simulink model "ABS"  (R2022b)
settings: Solver=VariableStepAuto  StartTime=0.0  StopTime=25  RelTol=1e-3
model workspace (MAT data in the model file):
  I = 5
  Jw = 0.02
  R = 0.28
  g = 9.81
  m = 75
  rw = 1.25
  v0 = 44
settings Model: Creator=ParkJunHo  LastModifiedBy=ParkJunHo

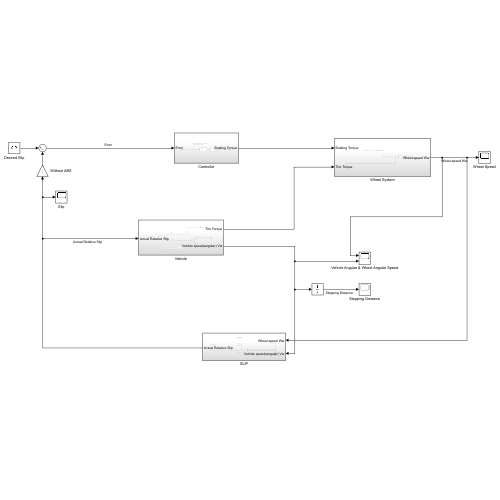
[thumbnail: Simulink's stored preview of the top-level diagram]
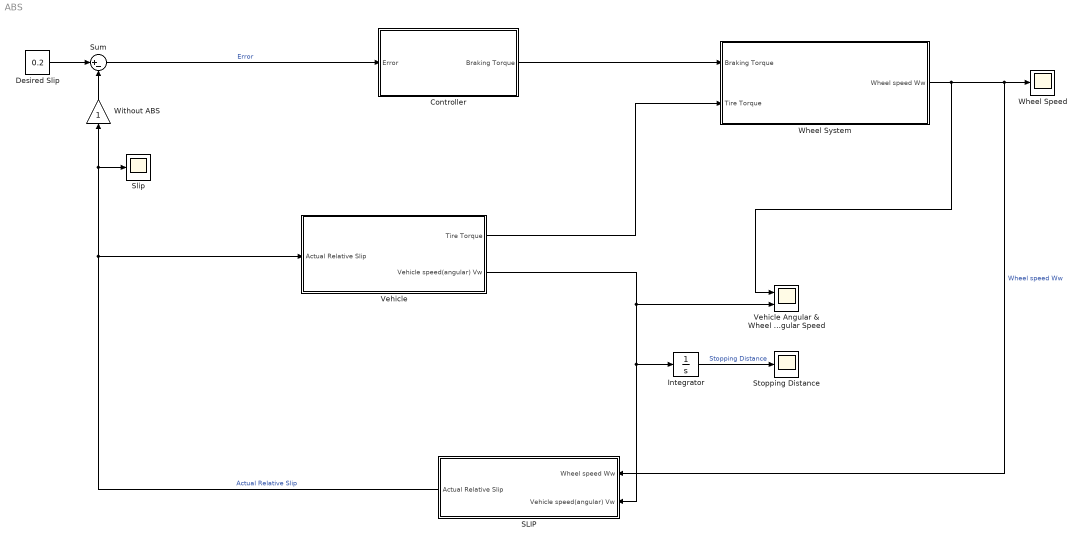
== system ABS ==
  Controller : Subsystem
  Desired Slip : Constant  Value=0.2
  Integrator : Integrator
  SLIP : Subsystem
  Slip : Scope
  Stopping Distance : Scope
  Sum : Sum  Inputs=|+-
  Vehicle : Subsystem
  Vehicle Angular & Wheel Angular Speed : Scope  NumInputPorts=2
  Wheel Speed : Scope
  Wheel System : Subsystem
  Without ABS : Gain
  wires:
  Desired Slip/1 -> Sum/1
  Wheel System/1(Wheel speed Ww) -> Vehicle Angular & Wheel Angular Speed/1, SLIP/1(Wheel speed Ww), Wheel Speed/1  "Wheel speed Ww"
  Sum/1 -> Controller/1(Error)  "Error"
  Controller/1(Braking Torque) -> Wheel System/1(Braking Torque)
  SLIP/1(Actual Relative Slip) -> Without ABS/1, Slip/1, Vehicle/1(Actual Relative Slip)  "Actual Relative Slip"
  Vehicle/1(Tire Torque) -> Wheel System/2(Tire Torque)
  Vehicle/2(Vehicle speed(angular) Vw) -> Vehicle Angular & Wheel Angular Speed/2, Integrator/1, SLIP/2(Vehicle speed(angular) Vw)
  Integrator/1 -> Stopping Distance/1  "Stopping Distance"
  Without ABS/1 -> Sum/2

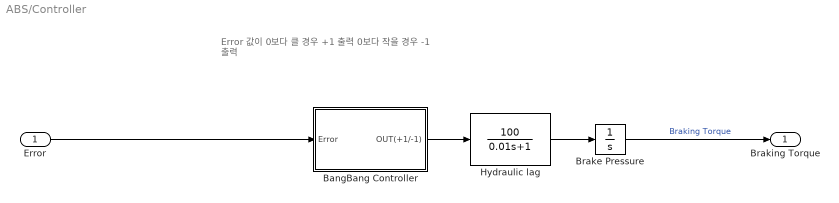
== system ABS/Controller ==
  note: Error 값이 0보다 클 경우 +1 출력
      | 0보다 작을 경우 -1 출력
  Error : Inport
  BangBang Controller : Subsystem
  Brake Pressure : Integrator  LimitOutput=on  UpperSaturationLimit=1000  LowerSaturationLimit=0
  Hydraulic lag : TransferFcn  Numerator=[100]  Denominator=[0.01 1]
  Braking Torque : Outport
  wires:
  BangBang Controller/1(OUT(+1/-1)) -> Hydraulic lag/1
  Hydraulic lag/1 -> Brake Pressure/1
  Error/1 -> BangBang Controller/1(Error)
  Brake Pressure/1 -> Braking Torque/1  "Braking Torque"

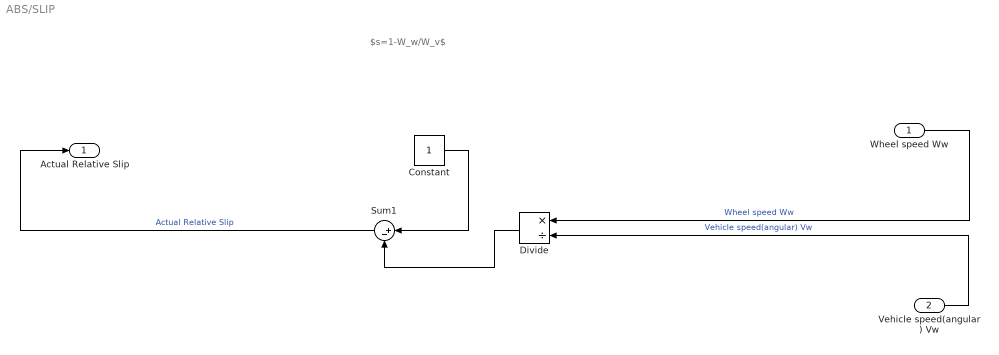
== system ABS/SLIP ==
  note: $s=1-W_w/W_v$
  Wheel speed Ww : Inport
  Vehicle speed(angular) Vw : Inport  Port=2
  Constant : Constant
  Divide : Product  Inputs=*/
  Sum1 : Sum  Inputs=|+-
  Actual Relative Slip : Outport
  wires:
  Divide/1 -> Sum1/2
  Wheel speed Ww/1 -> Divide/1  "Wheel speed Ww"
  Constant/1 -> Sum1/1
  Vehicle speed(angular) Vw/1 -> Divide/2  "Vehicle speed(angular) Vw"
  Sum1/1 -> Actual Relative Slip/1  "Actual Relative Slip"

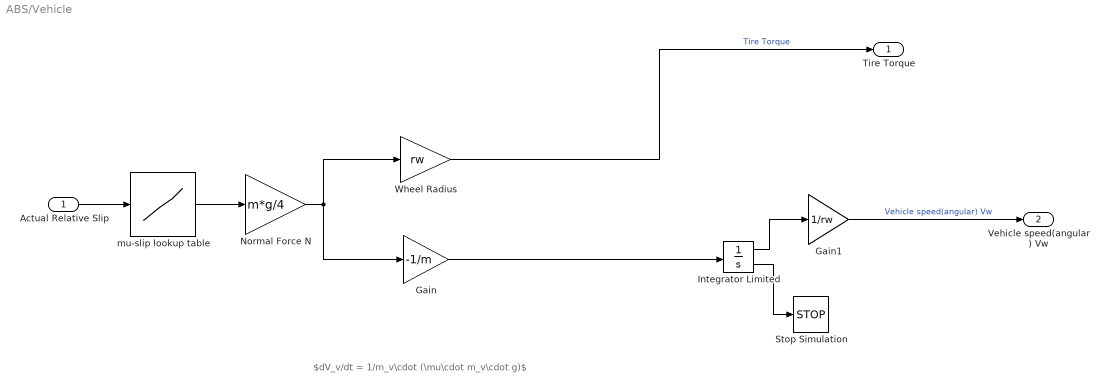
== system ABS/Vehicle ==
  note: $dV_v/dt = 1/m_v\cdot (\mu\cdot m_v\cdot g)$
  Actual Relative Slip : Inport
  Gain : Gain  Gain=-1/m
  Gain1 : Gain  Gain=1/rw
  Integrator Limited : Integrator  InitialCondition=v0  LimitOutput=on  UpperSaturationLimit=1000  LowerSaturationLimit=0  ShowSaturationPort=on
  Normal Force N : Gain  Gain=m*g/4
  Stop Simulation : Stop
  Wheel Radius : Gain  Gain=rw
  mu-slip lookup table : Lookup_n-D  NumberOfTableDimensions=1  BreakpointsForDimension1=[0,0.05,0.1,0.15,0.2,0.25,0.3,0.35,0.4,0.45,0.5,0.55,0.60,0.65,0.70,0.75,0.80,0.85,0.90,0.95,1]  Table=[0,0.4,0.8,0.97,1,0.98,0.96,0.94,0.92,0.9,0.88,0.855,0.83,0.81,0.79,0.77,0.75,0.73,0.72,0.71,0.7]  InternalRulePriority=Speed  RndMeth=Simplest
  Tire Torque : Outport
  Vehicle speed(angular) Vw : Outport  Port=2
  wires:
  Normal Force N/1 -> Gain/1, Wheel Radius/1
  Gain1/1 -> Vehicle speed(angular) Vw/1  "Vehicle speed(angular) Vw"
  Integrator Limited/2 -> Stop Simulation/1
  Wheel Radius/1 -> Tire Torque/1  "Tire Torque"
  mu-slip lookup table/1 -> Normal Force N/1
  Gain/1 -> Integrator Limited/1
  Integrator Limited/1 -> Gain1/1
  Actual Relative Slip/1 -> mu-slip lookup table/1

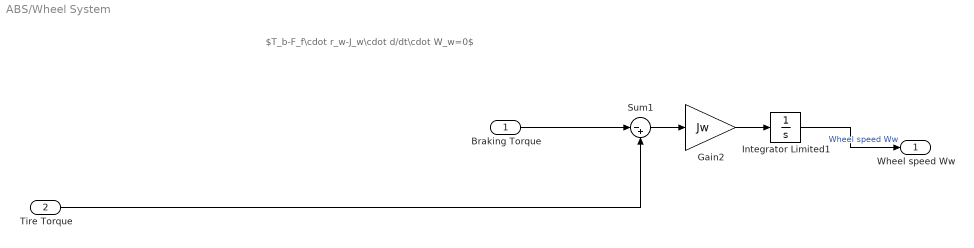
== system ABS/Wheel System ==
  note: $T_b-F_f\cdot r_w-J_w\cdot d/dt\cdot W_w=0$
  Braking Torque : Inport
  Tire Torque : Inport  Port=2
  Gain2 : Gain  Gain=Jw
  Integrator Limited1 : Integrator  InitialCondition=v0/rw  LimitOutput=on  UpperSaturationLimit=1000  LowerSaturationLimit=0
  Sum1 : Sum  Inputs=|-+
  Wheel speed Ww : Outport
  wires:
  Sum1/1 -> Gain2/1
  Gain2/1 -> Integrator Limited1/1
  Braking Torque/1 -> Sum1/1
  Integrator Limited1/1 -> Wheel speed Ww/1  "Wheel speed Ww"
  Tire Torque/1 -> Sum1/2

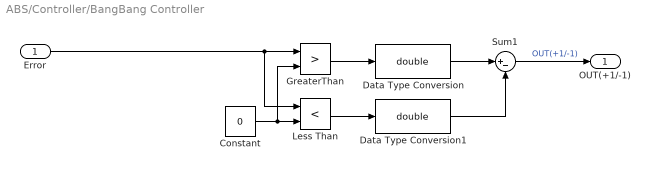
== system ABS/Controller/BangBang Controller ==
  Error : Inport
  Constant : Constant  Value=0
  Data Type Conversion : DataTypeConversion  OutDataTypeStr=double  SaturateOnIntegerOverflow=off
  Data Type Conversion1 : DataTypeConversion  OutDataTypeStr=double  SaturateOnIntegerOverflow=off
  GreaterThan : RelationalOperator  Operator=>  OutDataTypeStr=boolean  RndMeth=Simplest  InputSameDT=off
  Less Than : RelationalOperator  Operator=<  OutDataTypeStr=boolean  RndMeth=Simplest  InputSameDT=off
  Sum1 : Sum  Inputs=|+-
  OUT(+1/-1) : Outport
  wires:
  Less Than/1 -> Data Type Conversion1/1
  Constant/1 -> GreaterThan/2, Less Than/2
  GreaterThan/1 -> Data Type Conversion/1
  Data Type Conversion1/1 -> Sum1/2
  Error/1 -> Less Than/1, GreaterThan/1
  Sum1/1 -> OUT(+1/-1)/1  "OUT(+1/-1)"
  Data Type Conversion/1 -> Sum1/1
